simulink model "MFtest_1"  (R2016a)
settings: Solver=VariableStepAuto  StartTime=0.0  StopTime=10.0  RelTol=1e-3
values from neighbouring files (symbols this model uses):
  alpha = 0:0.025:0.2    [MFtest1.m]
  Fz1 = m*g*b/l    (= 6719.5301087)    [MFtest1.m]
  Fz2 = m*g*a/l    (= 8358.4398913)    [MFtest1.m]
settings Model: Creator=nnsyf  LastModifiedBy=nnsyf

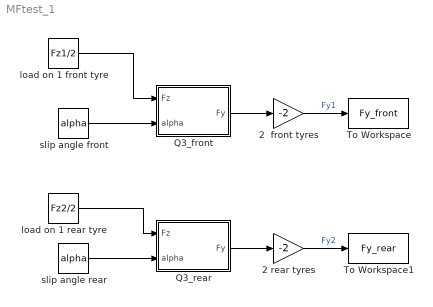
== system MFtest_1 ==
  2  front tyres : Gain  Gain=-2
  2 rear tyres : Gain  Gain=-2
  Q3_front : MATLAB Function  TreatAsAtomicUnit=on
  Q3_rear : MATLAB Function  TreatAsAtomicUnit=on
  To Workspace : ToWorkspace  VariableName=Fy_front  SampleTime=-1
      settings: Save2DSignal=2-D array (concatenate along first dimension)
  To Workspace1 : ToWorkspace  VariableName=Fy_rear  SampleTime=-1
      settings: Save2DSignal=2-D array (concatenate along first dimension)
  load on 1 front tyre : Constant  Value=Fz1/2
  load on 1 rear tyre : Constant  Value=Fz2/2
  slip angle front : Constant  Value=alpha
  slip angle rear : Constant  Value=alpha
  wires:
  slip angle front/1 -> Q3_front/2(alpha)
  slip angle rear/1 -> Q3_rear/2(alpha)
  Q3_front/1(Fy) -> 2  front tyres/1
  Q3_rear/1(Fy) -> 2 rear tyres/1
  2  front tyres/1 -> To Workspace/1  "Fy1"
  2 rear tyres/1 -> To Workspace1/1  "Fy2"
  load on 1 front tyre/1 -> Q3_front/1(Fz)
  load on 1 rear tyre/1 -> Q3_rear/1(Fz)

== matlab function MFtest_1/Q3_front ==
  data: Fz input; Fy output; alpha input
function Fy = fcn(Fz,alpha)

% Front lateral tyre force Fy[N] as function of tyre load Fz[N]and lteral slip angle alpha[rad]

Fy = Q3_front(Fz,alpha);

== matlab function MFtest_1/Q3_rear ==
  data: Fz input; Fy output; alpha input
function Fy = fcn(Fz,alpha)

% Rear lateral tyre force Fy[N] as function of tyre load Fz[N]and lteral slip angle alpha[rad]

Fy = Q3_rear(Fz,alpha);
